simulink model "torqueBalancingR2015a"  (Simulink 8.5)
settings: Solver=FixedStepDiscrete  StartTime=0.0  StopTime="CONFIG.SIMULATION_TIME "  FixedStep=CONFIG.Ts  RelTol=1e-3
InitFcn:
  | cd(fileparts(which(bdroot)));
  | initTorqueBalancing;
values from neighbouring files (symbols this model uses):
  WBT_robotName = 'iCub'    [initTorqueBalancing.m]
undefined symbols (not defined in the file or in its folder): bVectorConstraints, CONFIG, ConstraintsMatrix, DiscIntNeverNeededParam, gain, references, reg, ROBOT_DOF, ROBOT_DOF_FOR_SIMULINK, sat, SM, sm
libraries: WBToolboxLibrary x141, simulink x6
(part 4 of 4)

== matlab function Controller_QP/integralOf Hw/choose base to world transform ==
  data: lsole_H_root input double; w_H_b output double; rsole_H_root input double; constraints input double
function w_H_b = footOnGround(lsole_H_root,rsole_H_root,constraints)

    % A small state machine for choosing the base-to-world transform, according
    % to the foot on ground
    persistent w_H_fixedLink_intHw;

    if isempty(w_H_fixedLink_intHw) 
        w_H_fixedLink_intHw = eye(4);
    end
    
    w_H_b              = eye(4);
    toll               = 0.01;
    toll_W_H_fixedLink = 0.01;

    %% TWO FEET BALANCING AND LEFT FOOT BALANCING
    if constraints(1) >1-toll
        
        w_H_b      =  w_H_fixedLink_intHw * lsole_H_root;
    end
    
    %% RIGHT FOOT BALANCING 
    if  constraints(2) >1-toll
        
        % update w_H_fixedLink if it still assumes the left foot is the
        % fixed link
        checkIf_W_H_fixedLink_isTheIdentity = sum(diag(w_H_fixedLink_intHw))/4;
        
        if checkIf_W_H_fixedLink_isTheIdentity > 1-toll_W_H_fixedLink
            
             w_H_fixedLink_intHw   = w_H_fixedLink_intHw*lsole_H_root/rsole_H_root; % left foot is no longer a constraints
        end
        
        w_H_b       =  w_H_fixedLink_intHw*rsole_H_root;
    end
end

== matlab function Controller_QP/integralOf Hw/MATLAB Function ==
  data: qjErr input double; JL input double; JR input double; vbEquivalent output double; reg parameter double; activeFeetConstraints input double
 function vbEquivalent = generateReferencesForH(qjErr,JL,JR,reg,activeFeetConstraints)

    if activeFeetConstraints(1) == 1
    
        pinvJb       = (JL(:,1:6)'*JL(:,1:6) + reg.pinvDampVb*eye(6))\JL(:,1:6)';
        vbEquivalent = -pinvJb*JL(:,7:end)*qjErr;
    else
    
        pinvJb       = (JR(:,1:6)'*JR(:,1:6) + reg.pinvDampVb*eye(6))\JR(:,1:6)';
        vbEquivalent = -pinvJb*JR(:,7:end)*qjErr;
    end    
end

== matlab function State Machine/State machine walking/State Machine Walking/Compute w_H_b transform/from pos+quat to transfMatrix ==
  data: qt_fixed_LFoot input double; LFoot_is_active input double; w_H_fixed output double; qt_fixed_RFoot input double
function w_H_fixed = fromQuatToTransfMatrixFCN(qt_fixed_LFoot, LFoot_is_active, qt_fixed_RFoot)


    w_H_fixed = fromQuatToTransfMatrix(qt_fixed_LFoot, LFoot_is_active, qt_fixed_RFoot);
end

== matlab function State Machine/State machine walking/State Machine Walking/Compute w_H_b transform/w_H_root_link2/fromImuToHomogeousTransformFCN ==
  data: imu_H_link input double; imu_H_link_0 input double; link_H_root input double; inertial_0 input double; inertial input double; neck input double; w_H_root output double; CONFIG parameter double
function w_H_root = fromBaseToWorldWithImuFCN(imu_H_link,imu_H_link_0,link_H_root,inertial_0,inertial,neck,CONFIG)

    w_H_root = fromBaseToWorldWithImu(imu_H_link,imu_H_link_0,link_H_root,inertial_0,inertial,neck,CONFIG);
end

== matlab function Dump and visualize/plotNorms/norm2 ==
  data: u input double; normU output double
function normU = fcn(u)

    normU = norm(u);
end

== matlab function State Machine/State machine Yoga and Coordinator/State Machine Yoga/w_H_root_link2/fromImuToHomogeousTransformFCN ==
  data: imu_H_link input double; imu_H_link_0 input double; link_H_root input double; inertial_0 input double; inertial input double; neck input double; w_H_root output double; CONFIG parameter double
function w_H_root = fromBaseToWorldWithImuFCN(imu_H_link,imu_H_link_0,link_H_root,inertial_0,inertial,neck,CONFIG)

    w_H_root = fromBaseToWorldWithImu(imu_H_link,imu_H_link_0,link_H_root,inertial_0,inertial,neck,CONFIG);
end
